simulink model "Rotary_Inverted_Pendulum"  (R2020b)
settings: Solver=VariableStepAuto  StartTime=0.0  StopTime=60  RelTol=1e-3
settings Model: Creator=Taha  LastModifiedBy=Taha
settings DebuggingCC: UnderSpecifiedDimensionMsg=warning

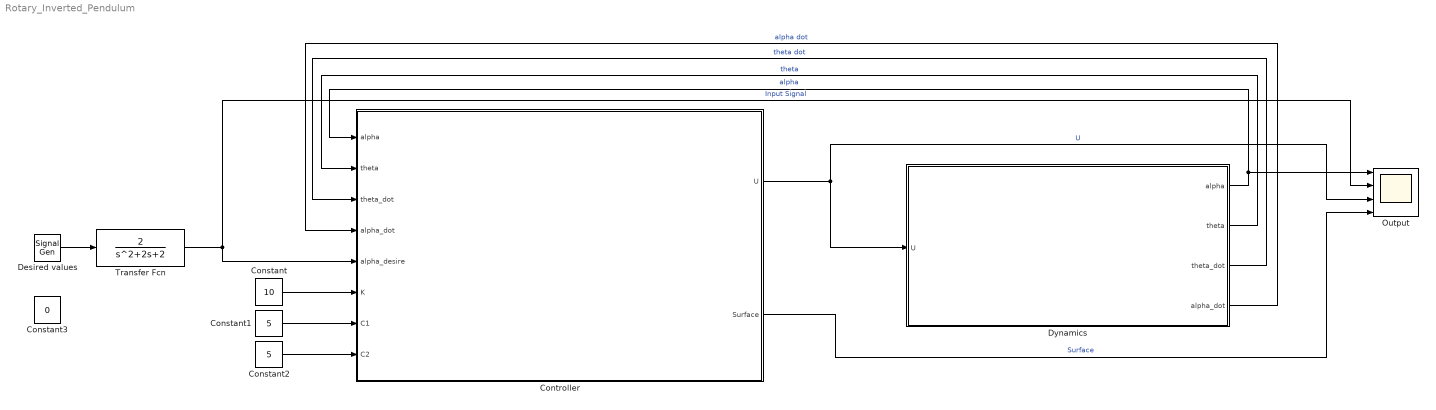
== system Rotary_Inverted_Pendulum ==
  Constant : Constant  Value=10
  Constant1 : Constant  Value=5
  Constant2 : Constant  Value=5
  Constant3 : Constant  Value=0
  Controller : Subsystem
  Desired values : SignalGenerator  Amplitude=0.5  Frequency=0.5  Units=rad/sec
  Dynamics : Subsystem
  Output : Scope  NumInputPorts=4
  Transfer Fcn : TransferFcn  Numerator=[2]  Denominator=[1 2 2]
  wires:
  Controller/1(U) -> Dynamics/1(U), Output/3  "U"
  Dynamics/1(alpha) -> Controller/1(alpha), Output/1  "alpha"
  Dynamics/2(theta) -> Controller/2(theta)  "theta"
  Dynamics/3(theta_dot) -> Controller/3(theta_dot)  "theta dot"
  Dynamics/4(alpha_dot) -> Controller/4(alpha_dot)  "alpha dot"
  Constant/1 -> Controller/6(K)
  Constant1/1 -> Controller/7(C1)
  Constant2/1 -> Controller/8(C2)
  Transfer Fcn/1 -> Output/2, Controller/5(alpha_desire)  "Input Signal"
  Controller/2(Surface) -> Output/4  "Surface"
  Desired values/1 -> Transfer Fcn/1

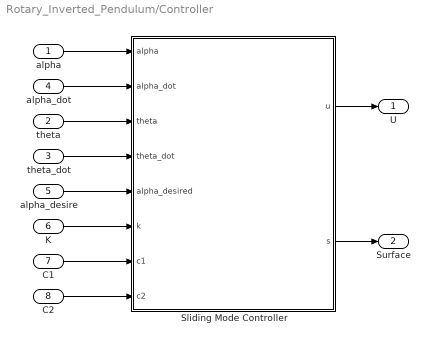
== system Rotary_Inverted_Pendulum/Controller ==
  alpha : Inport
  theta : Inport  Port=2
  theta_dot : Inport  Port=3
  alpha_dot : Inport  Port=4
  alpha_desire : Inport  Port=5
  K : Inport  Port=6
  C1 : Inport  Port=7
  C2 : Inport  Port=8
  Sliding Mode Controller : MATLAB Function  TreatAsAtomicUnit=on
  U : Outport
  Surface : Outport  Port=2
  wires:
  Sliding Mode Controller/1(u) -> U/1
  theta_dot/1 -> Sliding Mode Controller/4(theta_dot)
  alpha/1 -> Sliding Mode Controller/1(alpha)
  alpha_dot/1 -> Sliding Mode Controller/2(alpha_dot)
  theta/1 -> Sliding Mode Controller/3(theta)
  alpha_desire/1 -> Sliding Mode Controller/5(alpha_desired)
  K/1 -> Sliding Mode Controller/6(k)
  C1/1 -> Sliding Mode Controller/7(c1)
  C2/1 -> Sliding Mode Controller/8(c2)
  Sliding Mode Controller/2(s) -> Surface/1

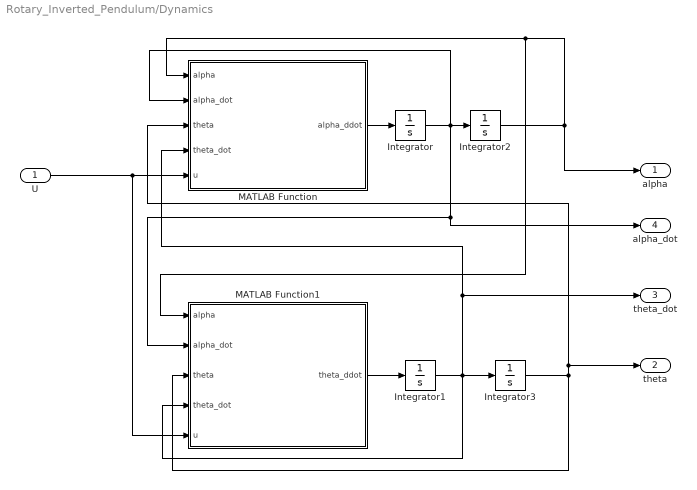
== system Rotary_Inverted_Pendulum/Dynamics ==
  U : Inport
  Integrator{,1..3} (4 alike) : Integrator  InitialCondition=randn
  MATLAB Function : MATLAB Function  TreatAsAtomicUnit=on
  MATLAB Function1 : MATLAB Function  TreatAsAtomicUnit=on
  alpha : Outport
  theta : Outport  Port=2
  theta_dot : Outport  Port=3
  alpha_dot : Outport  Port=4
  wires:
  U/1 -> MATLAB Function1/5(u), MATLAB Function/5(u)
  MATLAB Function/1(alpha_ddot) -> Integrator/1
  MATLAB Function1/1(theta_ddot) -> Integrator1/1
  Integrator/1 -> MATLAB Function1/2(alpha_dot), alpha_dot/1, Integrator2/1, MATLAB Function/2(alpha_dot)
  Integrator2/1 -> MATLAB Function1/1(alpha), MATLAB Function/1(alpha), alpha/1
  Integrator1/1 -> MATLAB Function/4(theta_dot), theta_dot/1, Integrator3/1, MATLAB Function1/4(theta_dot)
  Integrator3/1 -> theta/1, MATLAB Function/3(theta), MATLAB Function1/3(theta)

== matlab function Rotary_Inverted_Pendulum/Dynamics/MATLAB Function1 ==
  data: alpha input; alpha_dot input; theta input; theta_dot input; u input; theta_ddot output
function theta_ddot = compute_theta_ddot(alpha, alpha_dot, theta, theta_dot, u)
    % Constants (replace these with actual values)
   A = 3.291; % Replace with actual value
    B = 0.12519; % Replace with actual value
    C = 0.23688; % Replace with actual value
    D = 6.0521; % Replace with actual value
    E = 0.013201; % Replace with actual value
    F = 14.283; % Replace with actual value
    G = 1.4286; % Replace with actual value
    H = 1.72; % Replace with actual value
    I = 141.32; % Replace with actual value


    % Dynamics of theta_ddot
    fx_alpha = (-B^2 * alpha_dot * theta_dot * sin(2 * alpha) + ...
                B * C * alpha_dot^2 * sin(alpha) - ...
                0.5 * B * C * theta_dot^2 * sin(2 * alpha) * cos(alpha) - ...
                B * F * theta_dot - ...
                B * G * sign(theta_dot) - ... %..................................
                B * H * theta + ...
                C^2 * theta_dot * cos(alpha)^2 - ...
                0.5 * C * D * sin(2 * alpha) + ...
                C * E * alpha_dot * cos(alpha)) / ...
               (B * (A + B * sin(alpha)^2));

    gx_alpha = I / (A + B * sin(alpha)^2);

    alpha_ddot = fx_alpha + gx_alpha * u;

    f_theta = (-C * cos(alpha) * alpha_ddot + ...
               (C * sin(alpha)) * alpha_dot^2 - ...
               (2 * B * sin(alpha) * cos(alpha)) * alpha_dot * theta_dot - ...
               F * theta_dot - ...
               G * sign(theta_dot) - ...
               H * theta) / (A + B * sin(alpha)^2);

    g_theta = (I - C * cos(alpha) * gx_alpha) / (A + B * sin(alpha)^2);

    % Compute theta_ddot
    theta_ddot = f_theta + g_theta * u;
end

== matlab function Rotary_Inverted_Pendulum/Dynamics/MATLAB Function ==
  data: alpha input; alpha_dot input; theta input; theta_dot input; u input; alpha_ddot output
function alpha_ddot = compute_alpha_ddot(alpha, alpha_dot, theta, theta_dot, u)
    % Constants (replace these with actual values)
     A = 3.291; % Replace with actual value
    B = 0.12519; % Replace with actual value
    C = 0.23688; % Replace with actual value
    D = 6.0521; % Replace with actual value
    E = 0.013201; % Replace with actual value
    F = 14.283; % Replace with actual value
    G = 1.4286; % Replace with actual value
    H = 1.72; % Replace with actual value
    I = 141.32; % Replace with actual value

    % Dynamics of alpha_ddot
    fx_alpha = (-B^2 * alpha_dot * theta_dot * sin(2 * alpha) + ...
                B * C * alpha_dot^2 * sin(alpha) - ...
                0.5 * B * C * theta_dot^2 * sin(2 * alpha) * cos(alpha) - ...
                B * F * theta_dot - ...
                B * G * sign(theta_dot) - ...  %......................................................
                B * H * theta + ...
                C^2 * theta_dot * cos(alpha)^2 - ...
                0.5 * C * D * sin(2 * alpha) + ...
                C * E * alpha_dot * cos(alpha)) / ...
               (B * (A + B * sin(alpha)^2));

    gx_alpha = I / (A + B * sin(alpha)^2);

    % Compute alpha_ddot
    alpha_ddot = fx_alpha + gx_alpha * u;
end

== matlab function Rotary_Inverted_Pendulum/Controller/Sliding Mode Controller ==
  data: alpha input; u output; alpha_dot input; theta input; theta_dot input; alpha_desired input; k input; c1 input; c2 input; s output
function [u,s] = smc_controller(alpha, alpha_dot, theta, theta_dot, alpha_desired,k,c1,c2)
    % Controller parameters
    %c1 = 5; % Sliding surface coefficient
    %c2 = 5 ;
   % k = 8;  % Gain for SMC
    A = 3.291; % Replace with actual value
    B = 0.12519; % Replace with actual value
    C = 0.23688; % Replace with actual value
    D = 6.0521; % Replace with actual value
    E = 0.013201; % Replace with actual value
    F = 14.283; % Replace with actual value
    G = 1.4286; % Replace with actual value
    H = 1.72; % Replace with actual value
    I = 141.32; % Replace with actual value

	u = 0;
    % Sliding surface
    e = alpha - alpha_desired;
    s = c1 * e + c2 * alpha_dot;

    % Control law
    fx_alpha = (-B^2 * alpha_dot * theta_dot * sin(2 * alpha) + ...
                B * C * alpha_dot^2 * sin(alpha) - ...
                0.5 * B * C * theta_dot^2 * sin(2 * alpha) * cos(alpha) - ...
                B * F * theta_dot - ...
                B * G * sign(theta_dot) - ... %.........................................
                B * H * theta + ...
                C^2 * theta_dot * cos(alpha)^2 - ...
                0.5 * C * D * sin(2 * alpha) + ...
                C * E * alpha_dot * cos(alpha)) / ...
               (B * (A + B * sin(alpha)^2));
           
   gx_alpha = I / (A + B * sin(alpha)^2);

    u = -1 * (fx_alpha) / gx_alpha - (k / gx_alpha) * tanh(s);
end
